simulink model "proiect"  (R2022b)
settings: Solver=VariableStepAuto  StartTime=0.0  StopTime=50000.000  RelTol=1e-3
settings Model: Creator=ALex  LastModifiedBy=ALex

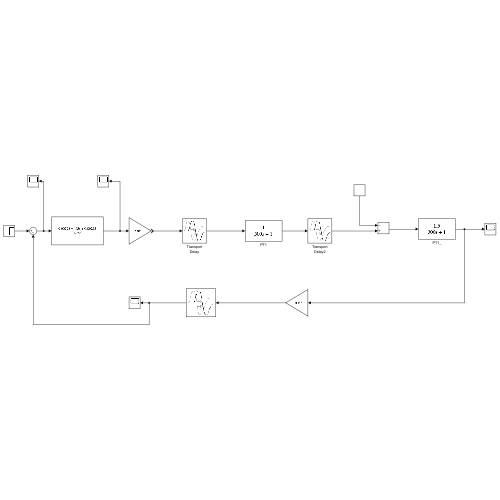
[thumbnail: Simulink's stored preview of the top-level diagram]
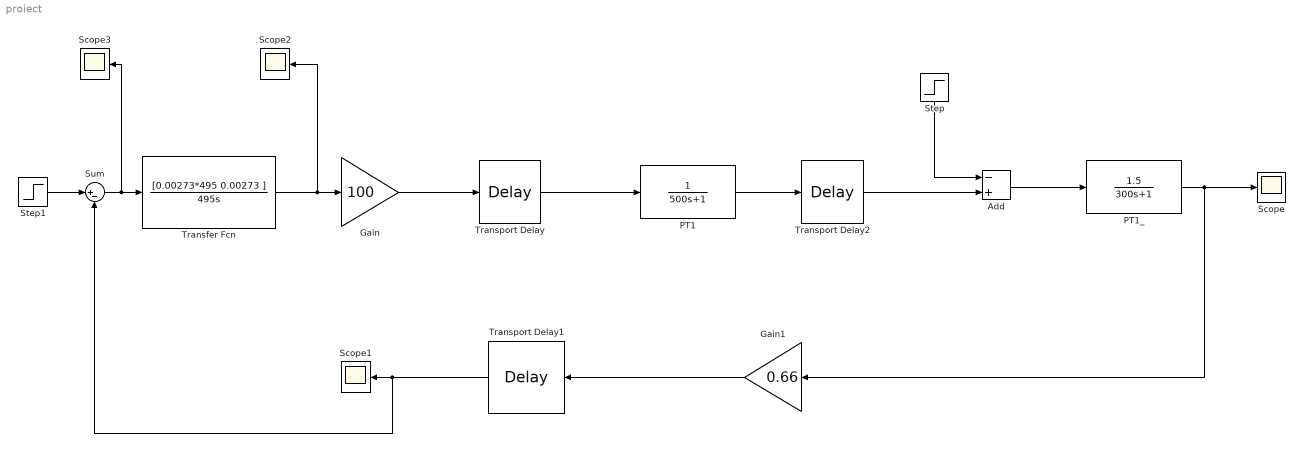
== system proiect ==
  Add : Sum  Inputs=-+
  Gain : Gain  Gain=100
  Gain1 : Gain  Gain=0.66
  PT1 : TransferFcn  Denominator=[500 1]
  PT1_ : TransferFcn  Numerator=[1.5]  Denominator=[300 1]
  Scope{,1..3} (4 alike) : Scope
  Step : Step  Time=20000  After=50  SampleTime=0
  Step1 : Step  Time=0  After=650  SampleTime=0
  Sum : Sum  Inputs=|+-
  Transfer Fcn : TransferFcn  Numerator=[0.00273*495 0.00273 ]  Denominator=[495 0]
  Transport Delay : TransportDelay  DelayTime=5
  Transport Delay1 : TransportDelay  DelayTime=20
  Transport Delay2 : TransportDelay  DelayTime=125
  wires:
  Gain/1 -> Transport Delay/1
  Transport Delay/1 -> PT1/1
  PT1/1 -> Transport Delay2/1
  Transport Delay2/1 -> Add/2
  Add/1 -> PT1_/1
  Gain1/1 -> Transport Delay1/1
  PT1_/1 -> Gain1/1, Scope/1
  Step1/1 -> Sum/1
  Transport Delay1/1 -> Sum/2, Scope1/1
  Sum/1 -> Scope3/1, Transfer Fcn/1
  Transfer Fcn/1 -> Scope2/1, Gain/1
  Step/1 -> Add/1
